simulink model "Unicycle_Robot_Dynamics"  (R2017b)
settings: Solver=VariableStepAuto  StartTime=0.0  StopTime=10.0  RelTol=1e-3
settings Model: Creator=Jesus  LastModifiedBy=Jesus

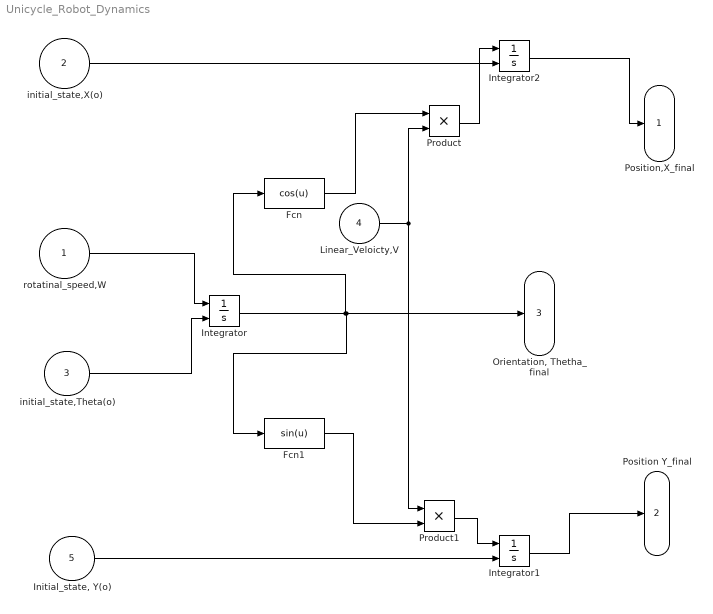
== system Unicycle_Robot_Dynamics ==
  "rotatinal_speed,W " : Inport
  "initial_state,X(o) " : Inport  Port=2
  "initial_state,Theta(o) " : Inport  Port=3
  "Linear_Veloicty,V " : Inport  Port=4
  "Initial_state, Y(o)" : Inport  Port=5
  Fcn : Fcn  Expr=cos(u)
  Fcn1 : Fcn  Expr=sin(u)
  Integrator : Integrator  InitialConditionSource=external
  Integrator1 : Integrator  InitialConditionSource=external
  Integrator2 : Integrator  InitialConditionSource=external
  Product : Product
  Product1 : Product
  "Position,X_final " : Outport
  "Position Y_final " : Outport  Port=2
  "Orientation, Thetha_final" : Outport  Port=3
  wires:
  "rotatinal_speed,W "/1 -> Integrator/1
  "initial_state,Theta(o) "/1 -> Integrator/2
  Integrator/1 -> "Orientation, Thetha_final"/1, Fcn1/1, Fcn/1
  Fcn/1 -> Product/1
  "Linear_Veloicty,V "/1 -> Product1/1, Product/2
  Product/1 -> Integrator2/1
  "initial_state,X(o) "/1 -> Integrator2/2
  Integrator2/1 -> "Position,X_final "/1
  "Initial_state, Y(o)"/1 -> Integrator1/2
  Fcn1/1 -> Product1/2
  Product1/1 -> Integrator1/1
  Integrator1/1 -> "Position Y_final "/1
